simulink library "ITKLib"  (R2022b)
settings: Solver=FixedStepDiscrete  StartTime=0.0  StopTime=10.0  FixedStep=0.01  RelTol=1e-3  EnableMultiTasking=on
values from neighbouring files (symbols this model uses):
  Glb_WhlRollgRd_SC = single(0.36)    [init_Global.m]
undefined symbols (not defined in the file or in its folder): docblock, SlDemoSign, SlDemoSign_Positive_SC, TaskTime_100ms_SC, TaskTime_10ms_SC, VehRefSpd_vMaxRefSpd_C
libraries: simulink x51, $bdroot x45, ITKLib_V14 x1
(part 8 of 10)

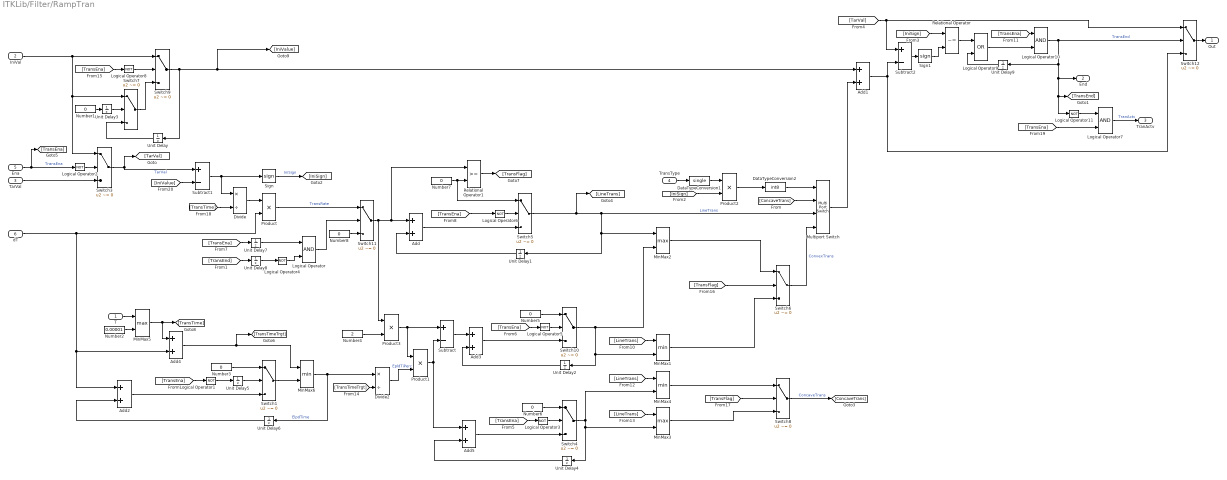
== system ITKLib/Filter/RampTran ==
  T : Inport
  IniVal : Inport  Port=2
  TarVal : Inport  Port=3
  TransType : Inport  Port=4
  Ena : Inport  Port=5
  dT : Inport  Port=6
  Add{,1..5} (6 alike) : Sum
  DataTypeConversion1 : DataTypeConversion  OutDataTypeStr=single  SaturateOnIntegerOverflow=off  RndMeth=Floor
  DataTypeConversion2 : DataTypeConversion  OutDataTypeStr=int8  SaturateOnIntegerOverflow=off  RndMeth=Floor
  Divide : Product  Inputs=*/
  Divide2 : Product  Inputs=*/
  Logical Operator : Logic  AllPortsSameDT=off  OutDataTypeStr=boolean
  Logical Operator{1..6,8,11} (8 alike) : Logic  Operator=NOT  AllPortsSameDT=off  OutDataTypeStr=boolean
  Logical Operator10 : Logic  AllPortsSameDT=off  OutDataTypeStr=boolean
  Logical Operator7 : Logic  AllPortsSameDT=off  OutDataTypeStr=boolean
  Logical Operator9 : Logic  Operator=OR  AllPortsSameDT=off  OutDataTypeStr=boolean
  MinMax1 : MinMax  Inputs=2
  MinMax2 : MinMax  Function=max  Inputs=2
  MinMax3 : MinMax  Function=max  Inputs=2
  MinMax4 : MinMax  Inputs=2
  MinMax5 : MinMax  Function=max  Inputs=2
  MinMax6 : MinMax  Inputs=2
  Multiport Switch : MultiPortSwitch  DataPortOrder=Specify indices  DataPortIndices={-1,0,1}  SaturateOnIntegerOverflow=off  InputSameDT=off
  Number1 : Constant  Value=0  OutDataTypeStr=boolean
      settings: AttributesFormatString=%<OutDataTypeStr>
  Number2 : Constant  Value=0.00001  OutDataTypeStr=single
      settings: AttributesFormatString=%<OutDataTypeStr>
  Number{3,5..8} (5 alike) : Constant  Value=0  OutDataTypeStr=single
      settings: AttributesFormatString=%<OutDataTypeStr>
  Number4 : Constant  Value=2  OutDataTypeStr=single
      settings: AttributesFormatString=%<OutDataTypeStr>
  Product{,1..3} (4 alike) : Product
  Relational Operator : RelationalOperator  Operator=~=  OutDataTypeStr=boolean  InputSameDT=off
  Relational Operator1 : RelationalOperator  OutDataTypeStr=boolean  InputSameDT=off
  Sign : Signum
  Sign1 : Signum
  Subtract : Sum  Inputs=+-
  Subtract1 : Sum  Inputs=+-
  Subtract2 : Sum  Inputs=+-
  Switch{1,3..12} (11 alike) : Switch  Criteria=u2 ~= 0  SaturateOnIntegerOverflow=off  InputSameDT=off
      settings: AttributesFormatString=Criteria : %<Criteria>
  Unit Delay{,1..2,4,6..9} (8 alike) : UnitDelay  SampleTime=-1  HasFrameUpgradeWarning=on
      settings: AttributesFormatString=<initial=%<X0>>
  Unit Delay3 : UnitDelay  InitialCondition=1  SampleTime=-1  HasFrameUpgradeWarning=on
      settings: AttributesFormatString=<initial=%<X0>>
  Unit Delay5 : UnitDelay  InitialCondition=1  SampleTime=-1  HasFrameUpgradeWarning=on
      settings: AttributesFormatString=<initial=%<X0>>
  Out : Outport
  End : Outport  Port=2
  TranActv : Outport  Port=3
  wires:
  Unit Delay9/1 -> Logical Operator9/2
  [TransEna] -> Logical Operator10/1
  Logical Operator9/1 -> Logical Operator10/2
  Relational Operator/1 -> Logical Operator9/1
  [IniSign] -> Product2/2
  TransType/1 -> DataTypeConversion1/1
  [TransEnd] -> Unit Delay8/1
  Logical Operator/1 -> Switch11/2
  Unit Delay7/1 -> Logical Operator/1
  Unit Delay8/1 -> Logical Operator4/1
  Switch1/1 -> MinMax6/2
  Logical Operator4/1 -> Logical Operator/2
  Unit Delay5/1 -> Switch1/2
  T/1 -> MinMax5/1
  Number2/1 -> MinMax5/2
  Switch7/1 -> Switch9/3
  Unit Delay/1 -> Switch7/3
  Unit Delay3/1 -> Switch7/2
  Number1/1 -> Unit Delay3/1
  Switch8/1 -> [ConcaveTrans]  "ConcaveTrans"
  MinMax3/1 -> Switch8/3
  MinMax4/1 -> Switch8/1
  Switch5/1 -> [LineTrans], Multiport Switch/3, MinMax2/1, Unit Delay1/1  "LineTrans"
  Switch4/1 -> MinMax3/2, Unit Delay4/1, MinMax4/2
  Relational Operator1/1 -> [TransFlag]
  Switch11/1 -> Relational Operator1/1, Add/1, Product3/1
  [TransEna] -> Logical Operator3/1
  Product1/1 -> Subtract/2, Add5/1
  Number6/1 -> Switch4/1
  Add5/1 -> Switch4/3
  Logical Operator3/1 -> Switch4/2
  Unit Delay4/1 -> Add5/2
  Divide2/1 -> Product1/2  "EpldTiPerc"
  MinMax1/1 -> Switch6/3
  Switch6/1 -> Multiport Switch/4  "ConvexTrans"
  MinMax2/1 -> Switch6/1
  Switch10/1 -> MinMax1/2, Unit Delay2/1, MinMax2/2
  [TransEna] -> Logical Operator5/1
  Subtract/1 -> Add3/1
  Number5/1 -> Switch10/1
  Add3/1 -> Switch10/3
  Logical Operator5/1 -> Switch10/2
  Unit Delay2/1 -> Add3/2
  Product3/1 -> Subtract/1, Product1/1
  [TransEna] -> Logical Operator1/1
  Logical Operator1/1 -> Unit Delay5/1
  MinMax6/1 -> Divide2/1, Unit Delay6/1  "ElpdTime"
  Number3/1 -> Switch1/1
  dT/1 -> Product/2, Add2/1, Add4/2
  Unit Delay6/1 -> Add2/2
  Add2/1 -> Switch1/3
  MinMax5/1 -> [TransTime], Add4/1
  Add4/1 -> [TransTimeTrgt], MinMax6/1
  [TransEna] -> Logical Operator6/1
  Logical Operator2/1 -> Switch3/2
  Logical Operator8/1 -> Switch9/2
  IniVal/1 -> Switch3/1, Switch7/1, Switch9/1
  Ena/1 -> [TransEna], Logical Operator2/1  "TransEna"
  Number8/1 -> Switch11/3
  Product/1 -> Switch11/1  "TransRate"
  [TransEna] -> Unit Delay7/1
  Switch9/1 -> [IniValue], Add1/1, Unit Delay/1
  TarVal/1 -> Switch3/3
  Switch12/1 -> Out/1
  [IniSign] -> Relational Operator/1
  Add1/1 -> Switch12/3, Subtract2/2
  Logical Operator10/1 -> Switch12/2, Logical Operator11/1, [TransEnd], End/1, Unit Delay9/1  "TransEnd"
  Subtract2/1 -> Sign1/1
  Sign1/1 -> Relational Operator/2
  [TarVal] -> Switch12/1, Subtract2/1
  Multiport Switch/1 -> Add1/2
  Number7/1 -> Switch5/1, Relational Operator1/2
  Add/1 -> Switch5/3
  Logical Operator6/1 -> Switch5/2
  Unit Delay1/1 -> Add/2
  Product2/1 -> DataTypeConversion2/1
  Subtract1/1 -> Sign/1, Divide/1
  Switch3/1 -> Subtract1/1, [TarVal]  "TarVal"
  Sign/1 -> [IniSign]  "IniSign"
  Divide/1 -> Product/1
  Number4/1 -> Product3/2
  [ConcaveTrans] -> Multiport Switch/2
  [LineTrans] -> MinMax1/1
  [LineTrans] -> MinMax4/1
  [LineTrans] -> MinMax3/1
  [TransTimeTrgt] -> Divide2/2
  [TransEna] -> Logical Operator8/1
  [TransFlag] -> Switch6/2
  [TransFlag] -> Switch8/2
  [TransTime] -> Divide/2
  [IniValue] -> Subtract1/2
  DataTypeConversion2/1 -> Multiport Switch/1
  [TransEna] -> Logical Operator7/2
  Logical Operator11/1 -> Logical Operator7/1
  Logical Operator7/1 -> TranActv/1  "TranActv"
  DataTypeConversion1/1 -> Product2/1

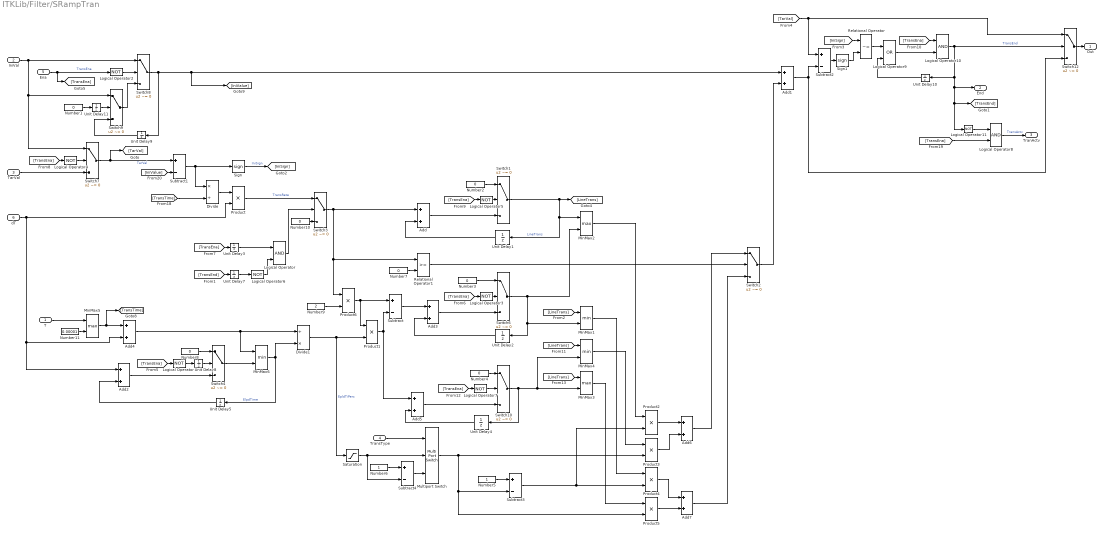
== system ITKLib/Filter/SRampTran ==
  T : Inport
  IniVal : Inport  Port=2
  TarVal : Inport  Port=3
  TransType : Inport  Port=4
  Ena : Inport  Port=5
  dT : Inport  Port=6
  Add{,1..7} (8 alike) : Sum
  Divide : Product  Inputs=*/
  Divide1 : Product  Inputs=/*
  Logical Operator : Logic  AllPortsSameDT=off  OutDataTypeStr=boolean
  Logical Operator{1..7,11} (8 alike) : Logic  Operator=NOT  AllPortsSameDT=off  OutDataTypeStr=boolean
  Logical Operator10 : Logic  AllPortsSameDT=off  OutDataTypeStr=boolean
  Logical Operator8 : Logic  AllPortsSameDT=off  OutDataTypeStr=boolean
  Logical Operator9 : Logic  Operator=OR  AllPortsSameDT=off  OutDataTypeStr=boolean
  MinMax1 : MinMax  Inputs=2
  MinMax2 : MinMax  Function=max  Inputs=2
  MinMax3 : MinMax  Function=max  Inputs=2
  MinMax4 : MinMax  Inputs=2
  MinMax5 : MinMax  Function=max  Inputs=2
  MinMax6 : MinMax  Inputs=2
  Multiport Switch : MultiPortSwitch  DataPortOrder=Specify indices  DataPortIndices={0,1}  SaturateOnIntegerOverflow=off  InputSameDT=off
  Number1 : Constant  Value=0  OutDataTypeStr=boolean
      settings: AttributesFormatString=%<OutDataTypeStr>
  Number{2..4,7..8,10} (6 alike) : Constant  Value=0  OutDataTypeStr=single
      settings: AttributesFormatString=%<OutDataTypeStr>
  Number11 : Constant  Value=0.00001  OutDataTypeStr=single
      settings: AttributesFormatString=%<OutDataTypeStr>
  Number5 : Constant  OutDataTypeStr=single
      settings: AttributesFormatString=%<OutDataTypeStr>
  Number6 : Constant  OutDataTypeStr=single
      settings: AttributesFormatString=%<OutDataTypeStr>
  Number9 : Constant  Value=2  OutDataTypeStr=single
      settings: AttributesFormatString=%<OutDataTypeStr>
  Product{,1..6} (7 alike) : Product
  Relational Operator : RelationalOperator  Operator=~=  OutDataTypeStr=boolean  InputSameDT=off
  Relational Operator1 : RelationalOperator  OutDataTypeStr=boolean  InputSameDT=off
  Saturation : Saturate  UpperLimit=1  LowerLimit=0
      settings: AttributesFormatString=<limits=%<UpperLimit>/%<LowerLimit>>
  Sign : Signum
  Sign1 : Signum
  Subtract{,1..4} (5 alike) : Sum  Inputs=+-
  Switch{1..4,6..10,12} (10 alike) : Switch  Criteria=u2 ~= 0  SaturateOnIntegerOverflow=off  InputSameDT=off
      Switch12 settings: AttributesFormatString=Criteria : %<Criteria>
      Switch2 settings: AttributesFormatString=Criteria : %<Criteria>
      Switch3 settings: AttributesFormatString=Criteria : %<Criteria>
      Switch4 settings: AttributesFormatString=Criteria : %<Criteria>
      Switch7 settings: AttributesFormatString=Criteria : %<Criteria>
      Switch8 settings: AttributesFormatString=Criteria : %<Criteria>
      Switch9 settings: AttributesFormatString=Criteria : %<Criteria>
  Unit Delay{1..5,7,9..10} (8 alike) : UnitDelay  SampleTime=-1  HasFrameUpgradeWarning=on
      settings: AttributesFormatString=<initial=%<X0>>
  Unit Delay11 : UnitDelay  InitialCondition=1  SampleTime=-1  HasFrameUpgradeWarning=on
      settings: AttributesFormatString=<initial=%<X0>>
  Unit Delay8 : UnitDelay  InitialCondition=1  SampleTime=-1  HasFrameUpgradeWarning=on
      settings: AttributesFormatString=<initial=%<X0>>
  Out : Outport
  End : Outport  Port=2
  TranActv : Outport  Port=3
  wires:
  Relational Operator/1 -> Logical Operator9/1
  Unit Delay10/1 -> Logical Operator9/2
  [TransEna] -> Logical Operator10/1
  Logical Operator9/1 -> Logical Operator10/2
  Number7/1 -> Relational Operator1/2
  [TransEnd] -> Unit Delay7/1
  Logical Operator6/1 -> Logical Operator/2
  Logical Operator/1 -> Switch3/2
  Unit Delay3/1 -> Logical Operator/1
  Unit Delay7/1 -> Logical Operator6/1
  Switch4/1 -> MinMax6/2
  Subtract4/1 -> Multiport Switch/3
  Number6/1 -> Subtract4/1
  Saturation/1 -> Multiport Switch/2, Subtract4/2
  Subtract3/1 -> Product4/2, Product2/2
  Number5/1 -> Subtract3/1
  Multiport Switch/1 -> Product3/2, Subtract3/2, Product5/2
  Product4/1 -> Add7/1
  Product5/1 -> Add7/2
  Product3/1 -> Add6/2
  Product2/1 -> Add6/1
  Add7/1 -> Switch2/3
  Add6/1 -> Switch2/1
  Divide1/1 -> Product1/2, Saturation/1  "EpldTiPerc"
  Relational Operator1/1 -> Switch2/2
  Divide/1 -> Product/1
  Sign/1 -> [IniSign]  "IniSign"
  Switch7/1 -> Subtract1/1, [TarVal]  "TarVal"
  Subtract1/1 -> Divide/1, Sign/1
  TransType/1 -> Multiport Switch/1
  Unit Delay1/1 -> Add/2
  Logical Operator5/1 -> Switch1/2
  Add/1 -> Switch1/3
  Number2/1 -> Switch1/1
  Switch2/1 -> Add1/2
  [TarVal] -> Subtract2/1, Switch12/1
  Sign1/1 -> Relational Operator/2
  Subtract2/1 -> Sign1/1
  Add1/1 -> Switch12/3, Subtract2/2
  [IniSign] -> Relational Operator/1
  Switch12/1 -> Out/1
  TarVal/1 -> Switch7/3
  Switch8/1 -> Unit Delay9/1, [IniValue], Add1/1
  [TransEna] -> Unit Delay3/1
  Product/1 -> Switch3/1  "TransRate"
  Number10/1 -> Switch3/3
  Ena/1 -> [TransEna], Logical Operator2/1  "TransEna"
  IniVal/1 -> Switch8/1, Switch7/1, Switch9/1
  Logical Operator2/1 -> Switch8/2
  [TransEna] -> Logical Operator4/1
  Logical Operator4/1 -> Switch7/2
  [TransEna] -> Logical Operator5/1
  Add4/1 -> MinMax6/1, Divide1/1
  MinMax5/1 -> [TransTime], Add4/1
  Add2/1 -> Switch4/3
  Unit Delay5/1 -> Add2/2
  dT/1 -> Product/2, Add4/2, Add2/1
  Number8/1 -> Switch4/1
  MinMax6/1 -> Unit Delay5/1, Divide1/2  "ElpdTime"
  Logical Operator1/1 -> Unit Delay8/1
  [TransEna] -> Logical Operator1/1
  Product6/1 -> Subtract/1, Product1/1
  Unit Delay2/1 -> Add3/2
  Logical Operator3/1 -> Switch6/2
  Add3/1 -> Switch6/3
  Number3/1 -> Switch6/1
  Subtract/1 -> Add3/1
  [TransEna] -> Logical Operator3/1
  Switch6/1 -> MinMax1/2, Unit Delay2/1, MinMax2/2
  MinMax2/1 -> Product2/1
  MinMax1/1 -> Product4/1
  Unit Delay4/1 -> Add5/2
  Logical Operator7/1 -> Switch10/2
  Add5/1 -> Switch10/3
  Number4/1 -> Switch10/1
  Product1/1 -> Add5/1, Subtract/2
  [TransEna] -> Logical Operator7/1
  Switch3/1 -> Add/1, Product6/1, Relational Operator1/1
  Switch10/1 -> Unit Delay4/1, MinMax3/2, MinMax4/2
  Switch1/1 -> Unit Delay1/1, MinMax2/1, [LineTrans]  "LineTrans"
  MinMax4/1 -> Product3/1
  MinMax3/1 -> Product5/1
  Number1/1 -> Unit Delay11/1
  Unit Delay11/1 -> Switch9/2
  Unit Delay9/1 -> Switch9/3
  Switch9/1 -> Switch8/3
  Number11/1 -> MinMax5/2
  T/1 -> MinMax5/1
  Unit Delay8/1 -> Switch4/2
  [IniValue] -> Subtract1/2
  Number9/1 -> Product6/2
  [TransTime] -> Divide/2
  [LineTrans] -> MinMax1/1
  [LineTrans] -> MinMax4/1
  [LineTrans] -> MinMax3/1
  Logical Operator11/1 -> Logical Operator8/1
  Logical Operator10/1 -> Switch12/2, Unit Delay10/1, Logical Operator11/1, [TransEnd], End/1  "TransEnd"
  [TransEna] -> Logical Operator8/2
  Logical Operator8/1 -> TranActv/1  "TransActv"

== system ITKLib/Filter/SecOrdBPF ==
  U : Inport
  Frq : Inport  Port=2
  Zeta : Inport  Port=3
  dT : Inport  Port=4
  DisableFilterDeal : Subsystem  TreatAsAtomicUnit=on
  Divide : Product  Inputs=**  OutDataTypeStr=single  RndMeth=Simplest
  Divide1 : Product  Inputs=*/  OutDataTypeStr=single  RndMeth=Simplest
  FilterJudgment : Subsystem
  If Action Subsystem : Subsystem  TreatAsAtomicUnit=on
  If1 : If  IfExpression=u1 ~=0
  Merge : Merge
  Unit Delay : UnitDelay  SampleTime=-1  HasFrameUpgradeWarning=on
  single1 : Constant  Value=6.2831852  OutDataTypeStr=single  SampleTime=-1
      settings: AttributesFormatString=%<OutDataTypeStr>
  single4 : Constant  OutDataTypeStr=single  SampleTime=-1
      settings: AttributesFormatString=%<OutDataTypeStr>
  y : Outport
  wires:
  dT/1 -> FilterJudgment/2(SampleTime), [SmpTime]
  Divide1/1 -> FilterJudgment/1(FilterTime)
  [In] -> If Action Subsystem/1(in)
  Divide/1 -> [Omega]
  If1/1 -> If Action Subsystem/Action
  Zeta/1 -> [Zeta]
  If Action Subsystem/1(FltOut) -> Merge/1
  Frq/1 -> Divide1/2, Divide/2
  single1/1 -> Divide/1
  single4/1 -> Divide1/1
  FilterJudgment/1(u1) -> If1/1
  [Omega] -> If Action Subsystem/3(Omega)
  If1/2 -> DisableFilterDeal/Action
  [FltOutLast] -> If Action Subsystem/2(FltOutOld)
  U/1 -> DisableFilterDeal/1(Input), [In]
  DisableFilterDeal/1(Output) -> Merge/2
  Unit Delay/1 -> [FltOutLast]
  [SmpTime] -> If Action Subsystem/5(SmpTime)
  Merge/1 -> Unit Delay/1, y/1
  [Zeta] -> If Action Subsystem/4(Zeta)

== system ITKLib/Hysteresis/HysteresisA ==
  R : Inport
  u : Inport  Port=2
  L : Inport  Port=3
  Logical Operator1 : Logic  Operator=OR  OutDataTypeStr=boolean
  Relational Operator : RelationalOperator  Operator=<=  OutDataTypeStr=boolean
  Relational Operator1 : RelationalOperator  Operator=<=  OutDataTypeStr=boolean
  Switch1 : Switch  Criteria=u2 ~= 0  SaturateOnIntegerOverflow=off  InputSameDT=off
      settings: AttributesFormatString=Criteria : %<Criteria>
  Unit Delay1 : UnitDelay  SampleTime=-1  HasFrameUpgradeWarning=on
      settings: AttributesFormatString=<initial=%<x0>>
  A : Outport
  wires:
  Logical Operator1/1 -> Switch1/2
  Relational Operator1/1 -> Switch1/1, Logical Operator1/1
  Relational Operator/1 -> Logical Operator1/2
  L/1 -> Relational Operator/2
  u/1 -> Relational Operator/1, Relational Operator1/2
  R/1 -> Relational Operator1/1
  Switch1/1 -> A/1, Unit Delay1/1
  Unit Delay1/1 -> Switch1/3

== system ITKLib/Hysteresis/HysteresisB ==
  R : Inport
  u : Inport  Port=2
  L : Inport  Port=3
  Number1 : Constant  OutDataTypeStr=boolean
      settings: AttributesFormatString=%<OutDataTypeStr>
  Number7 : Constant  Value=0  OutDataTypeStr=boolean
      settings: AttributesFormatString=%<OutDataTypeStr>
  Relational Operator : RelationalOperator  Operator=<=  OutDataTypeStr=boolean
  Relational Operator1 : RelationalOperator  OutDataTypeStr=boolean
  Switch2 : Switch  Criteria=u2 ~= 0  SaturateOnIntegerOverflow=off  InputSameDT=off
      settings: AttributesFormatString=Criteria : %<Criteria>
  Switch3 : Switch  Criteria=u2 ~= 0  SaturateOnIntegerOverflow=off  InputSameDT=off
      settings: AttributesFormatString=Criteria : %<Criteria>
  Unit Delay1 : UnitDelay  SampleTime=-1  HasFrameUpgradeWarning=on
      settings: AttributesFormatString=<initial=%<x0>>
  B : Outport
  wires:
  Switch3/1 -> Unit Delay1/1, B/1
  u/1 -> Relational Operator1/1, Relational Operator/1
  Relational Operator/1 -> Switch2/2
  Relational Operator1/1 -> Switch3/2
  L/1 -> Relational Operator/2
  Switch2/1 -> Switch3/3
  Number7/1 -> Switch3/1
  R/1 -> Relational Operator1/2
  Number1/1 -> Switch2/1
  Unit Delay1/1 -> Switch2/3

== system ITKLib/Limit/Limit ==
  MX : Inport
  u : Inport  Port=2
  MN : Inport  Port=3
  GreaterOrEqual : RelationalOperator  OutDataTypeStr=boolean
  MinMax : MinMax  Inputs=2  SaturateOnIntegerOverflow=on
  MinMax1 : MinMax  Function=max  Inputs=2  SaturateOnIntegerOverflow=on
  MinMax2 : MinMax  Function=max  Inputs=2  SaturateOnIntegerOverflow=on
  MinMax3 : MinMax  Inputs=2  SaturateOnIntegerOverflow=on
  Switch : Switch  Criteria=u2 ~= 0  SaturateOnIntegerOverflow=off  InputSameDT=off
      settings: AttributesFormatString=Criteria : %<Criteria>
  y : Outport  InitialOutput=0
  wires:
  MX/1 -> [MX], GreaterOrEqual/1
  u/1 -> [u], MinMax1/1
  MN/1 -> [MN], GreaterOrEqual/2
  MinMax1/1 -> MinMax/2
  Switch/1 -> y/1
  GreaterOrEqual/1 -> Switch/2
  MinMax/1 -> Switch/1
  [u] -> MinMax2/1
  [MX] -> MinMax2/2
  MinMax2/1 -> MinMax3/1
  [MN] -> MinMax3/2
  MinMax3/1 -> Switch/3
  [MN] -> MinMax1/2
  [MX] -> MinMax/1

== system ITKLib/Limit/LimitAndExcess ==
  MX : Inport
  u : Inport  Port=2
  MN : Inport  Port=3
  GreaterOrEqual : RelationalOperator  OutDataTypeStr=boolean
  MinMax2 : MinMax  Inputs=2  SaturateOnIntegerOverflow=on
  MinMax3 : MinMax  Function=max  Inputs=2  SaturateOnIntegerOverflow=on
  MinMax4 : MinMax  Function=max  Inputs=2  SaturateOnIntegerOverflow=on
  MinMax5 : MinMax  Inputs=2  SaturateOnIntegerOverflow=on
  Relational Operator1 : RelationalOperator  Operator=<  OutDataTypeStr=boolean
  Relational Operator4 : RelationalOperator  Operator=>  OutDataTypeStr=boolean
  Subtract : Sum  Inputs=+-
  Subtract1 : Sum  Inputs=+-
  Switch : Switch  Criteria=u2 ~= 0  SaturateOnIntegerOverflow=off  InputSameDT=off
      settings: AttributesFormatString=Criteria : %<Criteria>
  Switch2 : Switch  Criteria=u2 ~= 0  SaturateOnIntegerOverflow=off  InputSameDT=off
      settings: AttributesFormatString=Criteria : %<Criteria>
  Switch3 : Switch  Criteria=u2 ~= 0  SaturateOnIntegerOverflow=off  InputSameDT=off
      settings: AttributesFormatString=Criteria : %<Criteria>
  single : Constant  Value=0  OutDataTypeStr=single
      settings: AttributesFormatString=%<OutDataTypeStr>
  single1 : Constant  Value=0  OutDataTypeStr=single
      settings: AttributesFormatString=%<OutDataTypeStr>
  y : Outport  InitialOutput=0
  ExceUpLim : Outport  Port=2  InitialOutput=0
  ExceLowLim : Outport  Port=3  InitialOutput=0
  wires:
  Switch/1 -> y/1
  Subtract/1 -> Switch2/1, Relational Operator4/1
  Switch3/1 -> ExceLowLim/1
  [u] -> Subtract/1
  [u] -> Subtract1/1
  single/1 -> Relational Operator4/2, Switch2/3
  Relational Operator4/1 -> Switch2/2
  Switch2/1 -> ExceUpLim/1
  Relational Operator1/1 -> Switch3/2
  Subtract1/1 -> Relational Operator1/1, Switch3/1
  single1/1 -> Relational Operator1/2, Switch3/3
  [u] -> MinMax4/1
  [MX] -> MinMax2/1
  GreaterOrEqual/1 -> Switch/2
  MX/1 -> [MX], GreaterOrEqual/1
  MN/1 -> [MN], GreaterOrEqual/2
  MinMax3/1 -> MinMax2/2
  MinMax2/1 -> Switch/1
  u/1 -> [u], MinMax3/1
  MinMax4/1 -> MinMax5/1
  [MN] -> MinMax3/2
  [MN] -> MinMax5/2
  [MX] -> MinMax4/2
  MinMax5/1 -> Switch/3
  [MN] -> Subtract1/2
  [MX] -> Subtract/2

== system ITKLib/Limit/LimitAndFlag ==
  MX : Inport
  u : Inport  Port=2
  MN : Inport  Port=3
  AND : Logic  OutDataTypeStr=boolean
  GreaterOrEqual : RelationalOperator  OutDataTypeStr=boolean
  Logical Operator1 : Logic  Operator=NOT  AllPortsSameDT=off  OutDataTypeStr=boolean
  MinMax2 : MinMax  Inputs=2  SaturateOnIntegerOverflow=on
  MinMax3 : MinMax  Function=max  Inputs=2  SaturateOnIntegerOverflow=on
  MinMax4 : MinMax  Function=max  Inputs=2  SaturateOnIntegerOverflow=on
  MinMax5 : MinMax  Inputs=2  SaturateOnIntegerOverflow=on
  OR : Logic  Operator=OR  OutDataTypeStr=boolean
  Relational Operator : RelationalOperator  Operator=>  OutDataTypeStr=boolean
  Relational Operator1 : RelationalOperator  Operator=<  OutDataTypeStr=boolean
  Switch : Switch  Criteria=u2 ~= 0  SaturateOnIntegerOverflow=off  InputSameDT=off
      settings: AttributesFormatString=Criteria : %<Criteria>
  y : Outport  InitialOutput=0
  bMax : Outport  Port=2  InitialOutput=0
  bMin : Outport  Port=3  InitialOutput=0
  LimFlag : Outport  Port=4  InitialOutput=0
  wires:
  AND/1 -> bMin/1
  Logical Operator1/1 -> AND/2
  Relational Operator1/1 -> OR/2, AND/1
  Relational Operator/1 -> OR/1, Logical Operator1/1, bMax/1
  [u] -> Relational Operator/1
  [u] -> Relational Operator1/1
  [u] -> MinMax4/1
  [MX] -> MinMax2/1
  GreaterOrEqual/1 -> Switch/2
  MX/1 -> [MX], GreaterOrEqual/1
  MN/1 -> [MN], GreaterOrEqual/2
  MinMax3/1 -> MinMax2/2
  MinMax2/1 -> Switch/1
  u/1 -> [u], MinMax3/1
  MinMax4/1 -> MinMax5/1
  [MN] -> MinMax3/2
  [MN] -> MinMax5/2
  Switch/1 -> y/1
  [MX] -> MinMax4/2
  MinMax5/1 -> Switch/3
  [MX] -> Relational Operator/2
  [MN] -> Relational Operator1/2
  OR/1 -> LimFlag/1

== system ITKLib/Limit/LimitOnly ==
  Max : Inport
  u : Inport  Port=2
  Min : Inport  Port=3
  MinMax : MinMax  Inputs=2  SaturateOnIntegerOverflow=on
  MinMax1 : MinMax  Function=max  Inputs=2  SaturateOnIntegerOverflow=on
  y : Outport  InitialOutput=0
  wires:
  MinMax/1 -> y/1
  MinMax1/1 -> MinMax/2
  u/1 -> MinMax1/1
  Max/1 -> MinMax/1
  Min/1 -> MinMax1/2

== system ITKLib/Limit/UpdFac ==
  NewFac : Inport
  OldFac : Inport  Port=2
  NewFacSt : Inport  Port=3
  OldFacSt : Inport  Port=4
  Lower : RelationalOperator  Operator=<  OutDataTypeStr=boolean
  Switch : Switch  Criteria=u2 ~= 0  SaturateOnIntegerOverflow=off  InputSameDT=off
      settings: AttributesFormatString=Criteria : %<Criteria>
  Switch1 : Switch  Criteria=u2 ~= 0  SaturateOnIntegerOverflow=off  InputSameDT=off
      settings: AttributesFormatString=Criteria : %<Criteria>
  Fac : Outport
  FacSt : Outport  Port=2
  wires:
  OldFacSt/1 -> Switch1/3
  NewFacSt/1 -> Switch1/1
  Switch1/1 -> FacSt/1
  Switch/1 -> Fac/1
  Lower/1 -> Switch/2, [NewFacLoOldFac]
  OldFac/1 -> Lower/2, Switch/3
  NewFac/1 -> Lower/1, Switch/1
  [NewFacLoOldFac] -> Switch1/2

== system ITKLib/Limit/UpdMaxMin ==
  NewMax : Inport
  OldMax : Inport  Port=2
  NewMaxSt : Inport  Port=3
  OldMaxSt : Inport  Port=4
  NewMin : Inport  Port=5
  OldMin : Inport  Port=6
  NewMinSt : Inport  Port=7
  OldMinSt : Inport  Port=8
  Lower : RelationalOperator  Operator=<  OutDataTypeStr=boolean
  Lower1 : RelationalOperator  Operator=>  OutDataTypeStr=boolean
  Switch{,1..3} (4 alike) : Switch  Criteria=u2 ~= 0  SaturateOnIntegerOverflow=off  InputSameDT=off
      settings: AttributesFormatString=Criteria : %<Criteria>
  Max : Outport
  MaxSt : Outport  Port=2
  Min : Outport  Port=3
  MinSt : Outport  Port=4
  wires:
  NewMinSt/1 -> Switch3/1
  OldMinSt/1 -> Switch3/3
  Switch3/1 -> MinSt/1
  Switch2/1 -> Min/1
  Lower1/1 -> Switch2/2, [NewMinUpOldMin]
  OldMin/1 -> Lower1/2, Switch2/3
  NewMin/1 -> Lower1/1, Switch2/1
  OldMaxSt/1 -> Switch1/3
  NewMaxSt/1 -> Switch1/1
  Switch1/1 -> MaxSt/1
  Switch/1 -> Max/1
  Lower/1 -> Switch/2, [NewMaxLoOldMax]
  OldMax/1 -> Lower/2, Switch/3
  NewMax/1 -> Lower/1, Switch/1
  [NewMaxLoOldMax] -> Switch1/2
  [NewMinUpOldMin] -> Switch3/2

== system ITKLib/Memory/EdgeBi ==
  u : Inport  OutDataTypeStr=boolean
  Relational Operator : RelationalOperator  Operator=~=  OutDataTypeStr=boolean  RndMeth=Simplest
  Unit Delay2 : UnitDelay  SampleTime=-1  HasFrameUpgradeWarning=on
      settings: AttributesFormatString=<initial=%<x0>>
  y : Outport  OutDataTypeStr=boolean
  wires:
  Unit Delay2/1 -> Relational Operator/2
  Relational Operator/1 -> y/1
  u/1 -> Relational Operator/1, Unit Delay2/1

== system ITKLib/Memory/EdgeFalling ==
  u : Inport  OutDataTypeStr=boolean
  Logical Operator : Logic  AllPortsSameDT=off  OutDataTypeStr=boolean
  Logical Operator1 : Logic  Operator=NOT  AllPortsSameDT=off  OutDataTypeStr=boolean
  Unit Delay2 : UnitDelay  SampleTime=-1  HasFrameUpgradeWarning=on
      settings: AttributesFormatString=<initial=%<x0>>
  y : Outport  OutDataTypeStr=boolean
  wires:
  Logical Operator1/1 -> Logical Operator/1
  u/1 -> Logical Operator1/1, Unit Delay2/1
  Logical Operator/1 -> y/1
  Unit Delay2/1 -> Logical Operator/2

== system ITKLib/Memory/EdgeRising ==
  u : Inport  OutDataTypeStr=boolean
  Logical Operator : Logic  AllPortsSameDT=off  OutDataTypeStr=boolean
  Logical Operator1 : Logic  Operator=NOT  AllPortsSameDT=off  OutDataTypeStr=boolean
  Unit Delay2 : UnitDelay  SampleTime=-1  HasFrameUpgradeWarning=on
      settings: AttributesFormatString=<initial=%<x0>>
  y : Outport  OutDataTypeStr=boolean
  wires:
  Unit Delay2/1 -> Logical Operator1/1
  Logical Operator1/1 -> Logical Operator/2
  Logical Operator/1 -> y/1
  u/1 -> Logical Operator/1, Unit Delay2/1

== system ITKLib/Memory/RSLatch ==
  S : Inport  OutDataTypeStr=boolean
  R : Inport  Port=2  OutDataTypeStr=boolean
  Logical Operator1 : Logic  Operator=NOT  AllPortsSameDT=off  OutDataTypeStr=boolean
  Logical_Operator4 : Logic  AllPortsSameDT=off  OutDataTypeStr=boolean
  Logical_Operator5 : Logic  Operator=OR  AllPortsSameDT=off  OutDataTypeStr=boolean
  Unit Delay : UnitDelay  SampleTime=-1  HasFrameUpgradeWarning=on
      settings: AttributesFormatString=<initial=%<x0>>
  Q : Outport  OutDataTypeStr=boolean
  wires:
  S/1 -> Logical_Operator5/1
  R/1 -> Logical Operator1/1
  Logical_Operator5/1 -> Logical_Operator4/2
  Logical Operator1/1 -> Logical_Operator4/1
  Logical_Operator4/1 -> Unit Delay/1, Q/1
  Unit Delay/1 -> Logical_Operator5/2

== system ITKLib/PID/PIController ==
  Max : Inport
  Min : Inport  Port=2
  Kp : Inport  Port=3
  Ki : Inport  Port=4
  u : Inport  Port=5
  PreC : Inport  Port=6
  R : Inport  Port=7  OutDataTypeStr=boolean
  RV : Inport  Port=8
  dT : Inport  Port=9
  MinMax : MinMax  Inputs=2
  MinMax1 : MinMax  Function=max  Inputs=2
  MinMax2 : MinMax  Inputs=2
  MinMax3 : MinMax  Function=max  Inputs=2
  MinMax4 : MinMax  Inputs=2
  MinMax5 : MinMax  Function=max  Inputs=2
  Number3 : Constant  Value=0  OutDataTypeStr=single
      settings: AttributesFormatString=%<OutDataTypeStr>
  Number4 : Constant  Value=0  OutDataTypeStr=single
      settings: AttributesFormatString=%<OutDataTypeStr>
  Product : Product  Inputs=**  RndMeth=Zero
  Product1 : Product  Inputs=**  RndMeth=Zero
  Product2 : Product  Inputs=**  RndMeth=Zero
  Relational Operator1 : RelationalOperator  OutDataTypeStr=boolean  InputSameDT=off
  Relational Operator3 : RelationalOperator  Operator=<=  OutDataTypeStr=boolean  InputSameDT=off
  Sum : Sum  Inputs=+++
  Sum1 : Sum  Inputs=+-
  Sum2 : Sum  Inputs=+-
  Sum3 : Sum
  Switch1 : Switch  Criteria=u2 ~= 0  SaturateOnIntegerOverflow=off  InputSameDT=off
      settings: AttributesFormatString=Criteria : %<Criteria>
  Switch3 : Switch  Criteria=u2 ~= 0  SaturateOnIntegerOverflow=off  InputSameDT=off
      settings: AttributesFormatString=Criteria : %<Criteria>
  Switch4 : Switch  Criteria=u2 ~= 0  SaturateOnIntegerOverflow=off  InputSameDT=off
      settings: AttributesFormatString=Criteria : %<Criteria>
  Unit Delay : UnitDelay  SampleTime=-1  HasFrameUpgradeWarning=on
      settings: AttributesFormatString=<initial=%<X0>>
  UnitDelay : UnitDelay  SampleTime=-1  HasFrameUpgradeWarning=on
      settings: AttributesFormatString=<Initial=%<x0>>
  UnitDelay1 : UnitDelay  SampleTime=-1  HasFrameUpgradeWarning=on
      settings: AttributesFormatString=<Initial=%<x0>>
  y : Outport
  KiOut : Outport  Port=2
  KpOut : Outport  Port=3
  wires:
  Product/1 -> KpOut/1, Sum/2
  u/1 -> Product1/1, Product/2
  Kp/1 -> Product/1
  Ki/1 -> Product1/2
  Switch4/1 -> Sum3/1
  Switch1/1 -> Switch4/3
  MinMax3/1 -> Switch1/1
  Number4/1 -> MinMax3/2
  MinMax2/1 -> Switch4/1
  Number3/1 -> MinMax2/2
  Product2/1 -> Switch1/3, MinMax3/1, MinMax2/1
  Relational Operator1/1 -> [UpLimit]
  MinMax/1 -> y/1
  Min/1 -> [Min], MinMax1/1
  Max/1 -> [Max], MinMax/1
  dT/1 -> Product2/2
  Sum/1 -> Relational Operator3/1, Relational Operator1/1, MinMax1/2
  R/1 -> Switch3/2
  Product1/1 -> Product2/1
  Unit Delay/1 -> Sum3/2
  RV/1 -> Switch3/1
  Sum3/1 -> Switch3/3
  MinMax1/1 -> MinMax/2
  MinMax5/1 -> MinMax4/2
  Switch3/1 -> MinMax5/2
  MinMax4/1 -> KiOut/1, Unit Delay/1, Sum/3
  Sum1/1 -> MinMax5/1
  Sum2/1 -> MinMax4/1
  PreC/1 -> [PreC], Sum2/2, Sum1/2
  [Max] -> Relational Operator1/2
  Relational Operator3/1 -> [LowLimit]
  [LowLimit] -> UnitDelay/1
  UnitDelay/1 -> Switch1/2
  [UpLimit] -> UnitDelay1/1
  UnitDelay1/1 -> Switch4/2
  [Max] -> Sum2/1
  [Min] -> Sum1/1
  [PreC] -> Sum/1
  [Min] -> Relational Operator3/2

== system ITKLib/PID/PICtrlrWithLimFlg ==
  Max : Inport
  Min : Inport  Port=2
  KpOutMax : Inport  Port=3
  KpOutMin : Inport  Port=4
  Kp : Inport  Port=5
  Ki : Inport  Port=6
  u : Inport  Port=7
  PreC : Inport  Port=8
  R : Inport  Port=9  OutDataTypeStr=boolean
  RV : Inport  Port=10
  dT : Inport  Port=11
  MinMax : MinMax  Inputs=2
  MinMax1 : MinMax  Function=max  Inputs=2
  MinMax2 : MinMax  Inputs=2
  MinMax3 : MinMax  Function=max  Inputs=2
  MinMax4 : MinMax  Inputs=2
  MinMax5 : MinMax  Function=max  Inputs=2
  MinMax8 : $bdroot/PID/PICtrlrWithLimFlg/MinMax1  Function=max  Inputs=2  OutMin=[]  OutMax=[]  SampleTime=-1
  MinMax9 : $bdroot/PID/PICtrlrWithLimFlg/MinMax  Function=min  Inputs=2  OutMin=[]  OutMax=[]  SampleTime=-1
  Number3 : Constant  Value=0  OutDataTypeStr=single
      settings: AttributesFormatString=%<OutDataTypeStr>
  Number4 : Constant  Value=0  OutDataTypeStr=single
      settings: AttributesFormatString=%<OutDataTypeStr>
  Product : Product  Inputs=**  RndMeth=Zero
  Product1 : Product  Inputs=**  RndMeth=Zero
  Product2 : Product  Inputs=**  RndMeth=Zero
  Relational Operator1 : RelationalOperator  Operator=<=  OutDataTypeStr=boolean  InputSameDT=off
  Relational Operator3 : RelationalOperator  OutDataTypeStr=boolean  InputSameDT=off
  Sum : Sum  Inputs=+++
  Sum1 : Sum  Inputs=+-
  Sum2 : Sum  Inputs=+-
  Sum3 : Sum
  Switch1 : Switch  Criteria=u2 ~= 0  SaturateOnIntegerOverflow=off  InputSameDT=off
      settings: AttributesFormatString=Criteria : %<Criteria>
  Switch3 : Switch  Criteria=u2 ~= 0  SaturateOnIntegerOverflow=off  InputSameDT=off
      settings: AttributesFormatString=Criteria : %<Criteria>
  Switch4 : Switch  Criteria=u2 ~= 0  SaturateOnIntegerOverflow=off  InputSameDT=off
      settings: AttributesFormatString=Criteria : %<Criteria>
  Unit Delay : UnitDelay  SampleTime=-1  HasFrameUpgradeWarning=on
      settings: AttributesFormatString=<initial=%<X0>>
  UnitDelay : UnitDelay  SampleTime=-1  HasFrameUpgradeWarning=on
      settings: AttributesFormatString=<Initial=%<x0>>
  UnitDelay1 : UnitDelay  SampleTime=-1  HasFrameUpgradeWarning=on
      settings: AttributesFormatString=<Initial=%<x0>>
  y : Outport
  KiOut : Outport  Port=2
  KpOut : Outport  Port=3
  UpLimActv : Outport  Port=4
  LowLimActv : Outport  Port=5
  wires:
  [PreC] -> Sum/1
  [Min] -> Sum1/1
  [Max] -> Sum2/1
  UnitDelay1/1 -> Switch4/2
  [UpLimit] -> UnitDelay1/1
  UnitDelay/1 -> Switch1/2
  [LowLimit] -> UnitDelay/1
  PreC/1 -> [PreC], Sum2/2, Sum1/2
  Sum2/1 -> MinMax4/1
  Sum1/1 -> MinMax5/1
  MinMax4/1 -> Sum/3, Unit Delay/1, KiOut/1
  Switch3/1 -> MinMax5/2
  MinMax5/1 -> MinMax4/2
  MinMax1/1 -> MinMax/2
  Sum3/1 -> Switch3/3
  RV/1 -> Switch3/1
  Unit Delay/1 -> Sum3/2
  Product1/1 -> Product2/1
  R/1 -> Switch3/2
  Sum/1 -> Relational Operator1/1, Relational Operator3/1, MinMax1/2
  dT/1 -> Product2/2
  Max/1 -> MinMax/1, [Max]
  Min/1 -> MinMax1/1, [Min]
  MinMax/1 -> y/1
  Product2/1 -> MinMax2/1, MinMax3/1, Switch1/3
  Number3/1 -> MinMax2/2
  MinMax2/1 -> Switch4/1
  Number4/1 -> MinMax3/2
  MinMax3/1 -> Switch1/1
  Switch1/1 -> Switch4/3
  Switch4/1 -> Sum3/1
  Ki/1 -> Product1/2
  Kp/1 -> Product/1
  u/1 -> Product/2, Product1/1
  MinMax9/1 -> KpOut/1, Sum/2
  Relational Operator3/1 -> UpLimActv/1, [UpLimit]
  Relational Operator1/1 -> LowLimActv/1, [LowLimit]
  KpOutMin/1 -> MinMax8/2
  Product/1 -> MinMax8/1
  MinMax8/1 -> MinMax9/2
  KpOutMax/1 -> MinMax9/1
  [Max] -> Relational Operator3/2
  [Min] -> Relational Operator1/2

== system ITKLib/PID/PIGovernor ==
  Max : Inport
  Min : Inport  Port=2
  Kp : Inport  Port=3
  Ki : Inport  Port=4
  u : Inport  Port=5
  Ena : Inport  Port=6  OutDataTypeStr=boolean
  R : Inport  Port=7  OutDataTypeStr=boolean
  RV : Inport  Port=8
  Prec : Inport  Port=9
  dT : Inport  Port=10
  I : Subsystem
  P : Subsystem
  PILim : Subsystem
  PIOut : Outport
  POut : Outport  Port=2
  IOut : Outport  Port=3
  wires:
  R/1 -> I/7(R)
  RV/1 -> I/8(RV)
  dT/1 -> I/9(dT)
  P/1(KpOut) -> POut/1, PILim/2(KpOut)
  [Prec] -> I/2(PreC)
  Ena/1 -> [Ena], I/6(Ena)
  [Min] -> PILim/4(Min)
  PILim/1(PIOut) -> PIOut/1
  [Ena] -> PILim/6(Ena)
  I/1(KiOut) -> PILim/3(KiOut), IOut/1
  u/1 -> [u], P/1(u)
  Ki/1 -> I/5(Ki)
  Min/1 -> [Min], I/4(Min)
  [Max] -> PILim/5(Max)
  [u] -> I/1(u)
  Max/1 -> [Max], I/3(Max)
  Prec/1 -> PILim/1(Prec), [Prec]
  Kp/1 -> P/2(Kp)

== system ITKLib/Special/ControlAlgorithm ==
  note: BMS
  note: MCU
  AdrcCtrl : Subsystem  mask(AdrcCtrl){}
      mask help:
      | Self-immunity technology is a control technology developed on the basis of PID control and in conjunction with the theoretical advantages of modern control, in response to the deficiencies of classical PID control. Depending on the function in the controller, the self-immunity controller can be divided into: Tracking Differentiator  TD module, Nonlinear State Error Feedback Control  NLSEF module, and expansion state observer ESO module.
      |
      | input signals:
      | yTar - the target value of the controlled signal
      | y   - the actual value of the controlled signal
      | all the other input signals are calibration data.
      | r - the velocity factor
      | h - filter factor
      | Ts - integration factor, unit is s
      | DlyCnt - the delay counter of derivative module
      | ESO_Alpha1、ESO_Alpha2、ESO_Alpha3、ESO_Beta1、ESO_Beta2、ESO_Beta3: calibration data of ESO module
      | NLSEF_Alpha0、NLSEF_Alpha1、NLSEF_Alpha2、NLSEF_Beta0、NLSEF_Beta1、NLSEF_Beta2: calibration data of NLSEF module
      | b - system factor
      | dT - sample time, single data type, uint is s
      |
      | outputs:
      | u - the adrc control signal
      |
      | Simulink Custom Model Library, created by MCC.
      mask Display:
      | color('blue')
      | disp('\fontsize{16}ADRC', 'texmode', 'on')
      | color('green');
      | text(1,0,'ITK','horizontalAlignment','right','verticalAlignment','bottom');
  CholCalc : MATLAB Function  TreatAsAtomicUnit=on  mask(CholCalc){}
  Lgtd_Lat_Force : Subsystem  mask(Lgtd & Lat Force){}
      mask help: Calculate the longitudinal and lateral force of the wheel.
      mask Display:
      | color('blue')
      | disp('\fontsize{12}Lgtd & Lat Force', 'texmode', 'on')
      | color('green');
      | text(1,0,'ITK','horizontalAlignment','right','verticalAlignment','bottom');
  QrCalc : MATLAB Function  TreatAsAtomicUnit=on  mask(QrCalc){}
  RCCirtVolt : Subsystem  mask(RC Circuit to Target Voltage){}
      mask help: Implement discrete approximation for Randles equivalent circuit approximation of battery cell impedance
      mask Display:
      | color('blue')
      | disp('\fontsize{12} RC Circuit Voltage', 'texmode', 'on')
      | color('green');
      | text(1,0,'ITK','horizontalAlignment','right','verticalAlignment','bottom');
      | 
      | % port_label('input', 1, 'dVint_target')
      | % port_label('input', 2, 'ser_res')
      | % port_label('input', 3, 'rc_res')
      | % port_label('input', 4, 'rc_cap')
      | % port_label('input', 5, 'dt')
      | % port_label('input', 6, 'Vc_curr')
      | % port_label('output', 1, 'current')
  RCCritCurr : Subsystem  mask(RC Circuit Current){}
      mask help:
      | Rearrangement of 'Randles' RC electrical model to estimate a current that will
      | bring the cell voltage to a target limit after a given period of time.
      mask Display:
      | color('blue')
      | disp('\fontsize{12} RC Circuit Current', 'texmode', 'on')
      | color('green');
      | text(1,0,'ITK','horizontalAlignment','right','verticalAlignment','bottom');
      | 
      | % port_label('input', 1, 'dVint_target')
      | % port_label('input', 2, 'ser_res')
      | % port_label('input', 3, 'rc_res')
      | % port_label('input', 4, 'rc_cap')
      | % port_label('input', 5, 'dt')
      | % port_label('input', 6, 'Vc_curr')
      | % port_label('output', 1, 'current')
  SvdCalc : MATLAB Function  TreatAsAtomicUnit=on  mask(SvdCalc){}

== system ITKLib/Special/Diagramm Chapter ==
  EmptySubsystem : Subsystem

== system ITKLib/Special/Document ==
  note: 主动阻尼， 根 据电机转速的波动，在特定频率范围的转速波动幅度较大时， MCU 输出防抖转矩进行波动抑制，快速将转速波动抑制下来
  Abbreviations : simulink/Model-Wide Utilities/DocBlock  Tag=HideFromReport  DocumentType=RTF
  Calibration Hints : simulink/Model-Wide Utilities/DocBlock  Tag=HideFromReport  DocumentType=RTF
  DocBlock : simulink/Model-Wide Utilities/DocBlock  DocumentType=Text
      content=|
      | Type your documentation here
  Function description : simulink/Model-Wide Utilities/DocBlock  Tag=HideFromReport  DocumentType=RTF
  Hardware Condition : simulink/Model-Wide Utilities/DocBlock  Tag=HideFromReport  DocumentType=RTF
  MdlInfo : simulink/Model-Wide Utilities/Model Info  Frame=on  DisplayStringWithTags=|  HorizontalTextAlignment=Left  LeftAlignmentValue=0.02
      | <ModelName>: IdqAct
      | <Project>: Geely_MCU
      | <ModelVersion>: 1.0.0.0
      | <Creator>: MaoChongchong
      | <CreatedDate>: 2023 08 29 14:45
      | <Description>: actual current calculation
      | %<LastModifiedBy>
      | %<LastModificationDate>
  Physical Overview : simulink/Model-Wide Utilities/DocBlock  Tag=HideFromReport  DocumentType=RTF
  PolarionID : Subsystem  mask(PolarionID){ReqID=MCU-13815, ReqLink=https://polarion-epm.itk-engineering.de/polarion/#/project/Geely_MCU/workitem?id=MCU-13815}
      mask prompts: ReqID "PolarionID"; ReqLink "Polarion ID Link"
      mask help: Simulink Custom Model Library, created by MCC.
      mask DialogControl ReqOpenBtn Prompt: Open Polarion ID Link
      mask DialogControl ReqOpenBtn Callback:
      | reqLink = get_param(gcb,'ReqLink');
      | 
      | if(exist(reqLink,'file'))
      |     [filepath,name,ext] = fileparts(reqLink)
      |     set_param(gcb, 'ReqLink',  [name, ext]);
      |     open(reqLink);
      | else
      |     web(reqLink);
      | end;
      mask Display:
      | color('blue')
      | Description = get_param(gcb,'ReqId');
      | text(0.05,0.5,'Polarion ID:','horizontalAlignment','left','verticalAlignment','middle');
      | text(0.6,0.5,Description,'horizontalAlignment','left','verticalAlignment','middle');
      | 
      | color('green');
      | text(1,0,'ITK','horizontalAlignment','right','verticalAlignment','bottom');
  Unit detailed design : simulink/Model-Wide Utilities/DocBlock  Tag=HideFromReport  DocumentType=RTF

== system ITKLib/Special/HideInReport ==

== system ITKLib/Special/InlineDescription ==

== system ITKLib/Special/ReportWithParent ==
  note: Documentation
  Copyright : simulink/Model-Wide Utilities/Model Info  Tag=HideFromReport  Frame=on  DisplayStringWithTags=|  HorizontalTextAlignment=Left  LeftAlignmentValue=0.02
      | © Meta Motoren- und Energie- Technik GmbH
      | 
      | Model Version: %<ModelVersion>
      | Date: %<LastModificationDate>
  Detailed Function Description : simulink/Model-Wide Utilities/DocBlock  Tag=HideFromReport  DocumentType=Text
      content=|
      | No detailed function description available!
  HideInReport : $bdroot/Special/HideInReport  Tag=HideFromReport  Description=This Block hides the system and the included subsystems from the report generation.
  Hints for Application : simulink/Model-Wide Utilities/DocBlock  Tag=HideFromReport  DocumentType=Text
      content=|
      | No Hints for application available!
  InlineDescription : $bdroot/Special/InlineDescription  Tag=HideFromReport  Description=Effects that the subsystem is shown in the context of the parent subsystem  ShowInLibBrowser=0  RefreshPar=0

== system ITKLib/Special/RequirementDocumentation ==

== system ITKLib/Special/Revision History ==
  note: Documentation
  Copyright : simulink/Model-Wide Utilities/Model Info  Frame=on  DisplayStringWithTags=|  HorizontalTextAlignment=Left  LeftAlignmentValue=0.02
      | © ITK Engineering Technology (Wu Xi) Co., Ltd. (ITKC)
      | 
      | Model Version: %<ModelVersion>
      | Date: %<LastModificationDate>
  HideInReport : $bdroot/Special/HideInReport  Tag=HideFromReport  Description=This Block hides the system and the included subsystems from the report generation.
  InlineDescription : $bdroot/Special/InlineDescription  Tag=HideFromReport  Description=Subsystem to store the Revision History  ShowInLibBrowser=0  RefreshPar=0

== system ITKLib/TimeCounter/Accum ==
  In : Inport
  IncLim : Inport  Port=2
  Rst : Inport  Port=3
  IV : Inport  Port=4
  Add5 : Sum
  Add6 : Sum
  Add9 : Sum
  Delay8 : Delay  DelayLength=1  InitialConditionSource=Input port
      settings: InputPortMap=u0,p4
  Greater2 : RelationalOperator  Operator=>  OutDataTypeStr=boolean
  OR : Logic  Operator=OR  OutDataTypeStr=boolean
  Switch1 : Switch  Criteria=u2 ~= 0  SaturateOnIntegerOverflow=off  InputSameDT=off
  Switch10 : Switch  Criteria=u2 ~= 0  SaturateOnIntegerOverflow=off  InputSameDT=off
  Switch11 : Switch  Criteria=u2 ~= 0  SaturateOnIntegerOverflow=off  InputSameDT=off
  Unit Delay : UnitDelay  SampleTime=-1  HasFrameUpgradeWarning=on
      settings: AttributesFormatString=<initial=%<x0>>
  single1 : Constant  Value=0  OutDataTypeStr=single
      settings: AttributesFormatString=%<OutDataTypeStr>
  single6 : Constant  Value=0  OutDataTypeStr=single
      settings: AttributesFormatString=%<OutDataTypeStr>
  single8 : Constant  Value=0  OutDataTypeStr=single
      settings: AttributesFormatString=%<OutDataTypeStr>
  Out : Outport
  wires:
  Unit Delay/1 -> Add6/1
  [Rst] -> Switch1/2
  In/1 -> Add6/2
  OR/1 -> Switch11/2
  Switch10/1 -> Add5/1
  single6/1 -> Switch10/3
  Switch11/1 -> Unit Delay/1, Add9/1
  single1/1 -> Switch1/1
  Add6/1 -> Greater2/1, Switch11/3
  Switch1/1 -> Delay8/1, Add9/2
  single8/1 -> Switch11/1
  IV/1 -> Delay8/2
  Add9/1 -> Out/1
  Greater2/1 -> Switch10/2, OR/1
  IncLim/1 -> Greater2/2, [IncLim]
  Rst/1 -> [Rst], OR/2
  Delay8/1 -> Add5/2
  [IncLim] -> Switch10/1
  Add5/1 -> Switch1/3

== system ITKLib/TimeCounter/CountR ==
  E : Inport  OutDataTypeStr=boolean
  R : Inport  Port=2  OutDataTypeStr=boolean
  Add1 : Sum  AccumDataTypeStr=uint16  OutDataTypeStr=uint16
  Constant4 : Constant  Value=MAX  OutDataTypeStr=uint16  SampleTime=-1
  MinMax : MinMax  Inputs=2  OutDataTypeStr=uint16
  Number1 : Constant  OutDataTypeStr=uint16
      settings: AttributesFormatString=%<OutDataTypeStr>
  Number8 : Constant  Value=0  OutDataTypeStr=uint16
      settings: AttributesFormatString=%<OutDataTypeStr>
  Relational Operator1 : RelationalOperator  OutDataTypeStr=boolean  InputSameDT=off
  Saturation2 : Saturate  UpperLimit=uint16(65534)  LowerLimit=uint16(0)
      settings: AttributesFormatString=|
      | UpperLimit = %<UpperLimit>
      | LowLimit = %<LowerLimit>
  Switch : Switch  Criteria=u2 ~= 0  OutDataTypeStr=uint16  SaturateOnIntegerOverflow=off  InputSameDT=off
      settings: AttributesFormatString=Criteria : %<Criteria>
  Switch1 : Switch  Criteria=u2 ~= 0  OutDataTypeStr=uint16  SaturateOnIntegerOverflow=off  InputSameDT=off
      settings: AttributesFormatString=Criteria : %<Criteria>
  Unit Delay1 : UnitDelay  InitialCondition=uint16(0)  SampleTime=-1  HasFrameUpgradeWarning=on
      settings: AttributesFormatString=<initial=%<x0>>
  Unit Delay3 : UnitDelay  InitialCondition=uint16(0)  SampleTime=-1  HasFrameUpgradeWarning=on
      settings: AttributesFormatString=<initial=%<x0>>
  Out : Outport
  Cnt : Outport  Port=2
  wires:
  Switch/1 -> MinMax/1
  Number8/1 -> Switch/1
  Unit Delay3/1 -> Add1/1
  R/1 -> Switch/2
  E/1 -> Switch1/2
  Number1/1 -> Add1/2
  Add1/1 -> Switch1/1
  Switch1/1 -> Saturation2/1
  Constant4/1 -> Relational Operator1/2, MinMax/2
  Relational Operator1/1 -> Out/1
  Unit Delay1/1 -> Switch1/3
  MinMax/1 -> Relational Operator1/1, Unit Delay3/1, Unit Delay1/1, Cnt/1
  Saturation2/1 -> Switch/3

== system ITKLib/TimeCounter/CountRIV ==
  E : Inport  OutDataTypeStr=boolean
  R : Inport  Port=2  OutDataTypeStr=boolean
  IV : Inport  Port=3
  Add2 : Sum  AccumDataTypeStr=uint16  OutDataTypeStr=uint16
  Constant6 : Constant  Value=MAX  OutDataTypeStr=uint16  SampleTime=-1
  MinMax1 : MinMax  Inputs=2  OutDataTypeStr=uint16
  Number1 : Constant  Value=0  OutDataTypeStr=boolean
      settings: AttributesFormatString=%<OutDataTypeStr>
  Number8 : Constant  OutDataTypeStr=uint16
      settings: AttributesFormatString=%<OutDataTypeStr>
  Relational Operator2 : RelationalOperator  OutDataTypeStr=boolean  InputSameDT=off
  Saturation2 : Saturate  UpperLimit=uint16(65534)  LowerLimit=uint16(0)
      settings: AttributesFormatString=|
      | UpperLimit = %<UpperLimit>
      | LowLimit = %<LowerLimit>
  Switch : Switch  Criteria=u2 ~= 0  OutDataTypeStr=uint16  SaturateOnIntegerOverflow=off  InputSameDT=off
      settings: AttributesFormatString=Criteria : %<Criteria>
  Switch4 : Switch  Criteria=u2 ~= 0  OutDataTypeStr=uint16  SaturateOnIntegerOverflow=off  InputSameDT=off
      settings: AttributesFormatString=Criteria : %<Criteria>
  Switch5 : Switch  Criteria=u2 ~= 0  OutDataTypeStr=uint16  SaturateOnIntegerOverflow=off  InputSameDT=off
      settings: AttributesFormatString=Criteria : %<Criteria>
  Unit Delay4 : UnitDelay  InitialCondition=uint16(0)  SampleTime=-1  HasFrameUpgradeWarning=on
      settings: AttributesFormatString=<initial=%<x0>>
  UnitDelay : UnitDelay  InitialCondition=1  SampleTime=-1  HasFrameUpgradeWarning=on
      settings: AttributesFormatString=<Initial=%<x0>>
  Out : Outport
  Cnt : Outport  Port=2
  wires:
  Unit Delay4/1 -> Add2/1, Switch4/3
  MinMax1/1 -> Relational Operator2/1, Switch5/3
  Switch/1 -> MinMax1/1
  Switch4/1 -> Saturation2/1
  IV/1 -> Switch5/1, Switch/1
  Constant6/1 -> Relational Operator2/2, MinMax1/2
  Number8/1 -> Add2/2
  Relational Operator2/1 -> Out/1
  E/1 -> Switch4/2
  R/1 -> Switch/2
  Add2/1 -> Switch4/1
  Switch5/1 -> Unit Delay4/1, Cnt/1
  Number1/1 -> UnitDelay/1
  UnitDelay/1 -> Switch5/2
  Saturation2/1 -> Switch/3
